simulink model "mrefrobotarm_modified_previous_y_previous_u_previous_ref_cover"  (R2018b)
settings: Solver=FixedStepAuto  StartTime=0.0  StopTime=20  RelTol=1e-3  AbsTol=1e-6
undefined symbols (not defined in the file or in its folder): cc, options
libraries: neural x396, simulink x1
(part 7 of 15)

== system mrefrobotarm_modified_previous_y_previous_u_previous_ref_cover/cov_error/Layer 3/Delays 1 ==
  "p{3}" : Inport  PortDimensions=30
      mask Display: e = 0.06;c1 = [120 230 180]/255;c2 = ([120 230 180]+0)/(256+128);c3 = ([120 230 180]+128)/(256+128);patch([0 1 1 0],[0 0 1 1],c1);patch([0 1 1 1-e 1-e 0+e],[0 0 1 1-e 0+e 0+e],c2);patch([0 0 1 1-e 0+e 0+e],[0 1 1 1-e 1-e 0+e],c3);plot([0 1 1 0 0],[0 0 1 1 0]);
  mux : Mux  Inputs=1
      mask Display: e = 0.06;c1 = [120 150 230]/255;c2 = ([120 150 230]+0)/383;c3 = ([120 150 230]+128)/383;patch([0 1 1 0],[0 0 1 1],c1);patch([0 1 1 1-e 1-e 0+e],[0 0 1 1-e 0+e 0+e],c2);patch([0 0 1 1-e 0+e 0+e],[0 1 1 1-e 1-e 0+e],c3);plot([0 1 1 0 0],[0 0 1 1 0]);disp('Mux')
  "pd{3,2}" : Outport
      mask Display: e = 0.06;c1 = [120 230 180]/255;c2 = ([120 230 180]+0)/(256+128);c3 = ([120 230 180]+128)/(256+128);patch([0 1 1 0],[0 0 1 1],c1);patch([0 1 1 1-e 1-e 0+e],[0 0 1 1-e 0+e 0+e],c2);patch([0 0 1 1-e 0+e 0+e],[0 1 1 1-e 1-e 0+e],c3);plot([0 1 1 0 0],[0 0 1 1 0]);
  wires:
  "p{3}"/1 -> mux/1
  mux/1 -> "pd{3,2}"/1

== system mrefrobotarm_modified_previous_y_previous_u_previous_ref_cover/cov_error/Layer 3/LW{3,2} ==
  "ad{3,2}" : Inport  PortDimensions=30
      mask Display: e = 0.06;c1 = [120 230 180]/255;c2 = ([120 230 180]+0)/(256+128);c3 = ([120 230 180]+128)/(256+128);patch([0 1 1 0],[0 0 1 1],c1);patch([0 1 1 1-e 1-e 0+e],[0 0 1 1-e 0+e 0+e],c2);patch([0 0 1 1-e 0+e 0+e],[0 1 1 1-e 1-e 0+e],c3);plot([0 1 1 0 0],[0 0 1 1 0]);
  "IW{3,2}(1,:)'" : Constant  Value=[-0.36344223341268999671882511393050663173198699951171875;-0.165155178341810537911982237346819601953029632568359375;0.347615078105802999264284380842582322657108306884765625;-0.30164554186513037326022868001018650829792022705078125;0.2759975456345065136787297888076864182949066162109375;0.2465662292665131427593649959817412309348583221435546875;0.1610224607061102319871537247308879159390926361083984375;-0.1798407133675627711522082563533331267535686492919921875;0.401376049002902191009667376420111395418643951416015625;-0.255050273303427832427558996641892008483409881591796875;0.352349460376939038752652777475304901599884033203125;-0.28687203005856043436239133370690979063510894775390625;-0.1992546066370121937705306436328100971877574920654296875;0.233402441264629001427266530299675650894641876220703125;-0.351246745396703807795546481429482810199260711669921875;-0.27181918807968930007490371281164698302745819091796875;0.2299774014947667810648823660812922753393650054931640625;0.283190968807739140711277059381245635449886322021484375;-0.2497764015090132849739035236780182458460330963134765625;-0.27863248514163230229456758024753071367740631103515625;0.37793893813860679475880033351131714880466461181640625;0.3335131904309964756549788944539614021778106689453125;-0.1504481789124049451178422032171511091291904449462890625;0.2409347112974611626601273428605054505169391632080078125;0.1106042034418963371233957104777800850570201873779296875;0.18259052723765833992075613423367030918598175048828125;-0.178194964093014274197912527597509324550628662109375;-0.232453072978504204915140007869922555983066558837890625;0.12259425656011870009454156615902320481836795806884765625;-0.295313678958903758076104395513539202511310577392578125]
      mask Display: e = 0.06;c1 = [120 150 230]/255;c2 = ([120 150 230]+0)/383;c3 = ([120 150 230]+128)/383;patch([0 1 1 0],[0 0 1 1],c1);patch([0 1 1 1-e 1-e 0+e],[0 0 1 1-e 0+e 0+e],c2);patch([0 0 1 1-e 0+e 0+e],[0 1 1 1-e 1-e 0+e],c3);plot([0 1 1 0 0],[0 0 1 1 0]);disp('weights');
  Mux : Mux  Inputs=1
      mask Display: e = 0.06;c1 = [120 150 230]/255;c2 = ([120 150 230]+0)/383;c3 = ([120 150 230]+128)/383;patch([0 1 1 0],[0 0 1 1],c1);patch([0 1 1 1-e 1-e 0+e],[0 0 1 1-e 0+e 0+e],c2);patch([0 0 1 1-e 0+e 0+e],[0 1 1 1-e 1-e 0+e],c3);plot([0 1 1 0 0],[0 0 1 1 0]);disp('Mux');
  dotprod1 : neural/Weight Functions/dotprod
  "lz{3,2}" : Outport
      mask Display: e = 0.06;c1 = [120 230 180]/255;c2 = ([120 230 180]+0)/(256+128);c3 = ([120 230 180]+128)/(256+128);patch([0 1 1 0],[0 0 1 1],c1);patch([0 1 1 1-e 1-e 0+e],[0 0 1 1-e 0+e 0+e],c2);patch([0 0 1 1-e 0+e 0+e],[0 1 1 1-e 1-e 0+e],c3);plot([0 1 1 0 0],[0 0 1 1 0]);
  wires:
  "IW{3,2}(1,:)'"/1 -> dotprod1/1
  "ad{3,2}"/1 -> dotprod1/2
  dotprod1/1 -> Mux/1
  Mux/1 -> "lz{3,2}"/1

== system mrefrobotarm_modified_previous_y_previous_u_previous_ref_cover/cov_no_error/Layer 1/Delays 1 ==
  "p{1}" : Inport  PortDimensions=10
      mask Display: e = 0.06;c1 = [120 230 180]/255;c2 = ([120 230 180]+0)/(256+128);c3 = ([120 230 180]+128)/(256+128);patch([0 1 1 0],[0 0 1 1],c1);patch([0 1 1 1-e 1-e 0+e],[0 0 1 1-e 0+e 0+e],c2);patch([0 0 1 1-e 0+e 0+e],[0 1 1 1-e 1-e 0+e],c3);plot([0 1 1 0 0],[0 0 1 1 0]);
  mux : Mux  Inputs=1
      mask Display: e = 0.06;c1 = [120 150 230]/255;c2 = ([120 150 230]+0)/383;c3 = ([120 150 230]+128)/383;patch([0 1 1 0],[0 0 1 1],c1);patch([0 1 1 1-e 1-e 0+e],[0 0 1 1-e 0+e 0+e],c2);patch([0 0 1 1-e 0+e 0+e],[0 1 1 1-e 1-e 0+e],c3);plot([0 1 1 0 0],[0 0 1 1 0]);disp('Mux')
  "pd{1,1}" : Outport
      mask Display: e = 0.06;c1 = [120 230 180]/255;c2 = ([120 230 180]+0)/(256+128);c3 = ([120 230 180]+128)/(256+128);patch([0 1 1 0],[0 0 1 1],c1);patch([0 1 1 1-e 1-e 0+e],[0 0 1 1-e 0+e 0+e],c2);patch([0 0 1 1-e 0+e 0+e],[0 1 1 1-e 1-e 0+e],c3);plot([0 1 1 0 0],[0 0 1 1 0]);
  wires:
  "p{1}"/1 -> mux/1
  mux/1 -> "pd{1,1}"/1

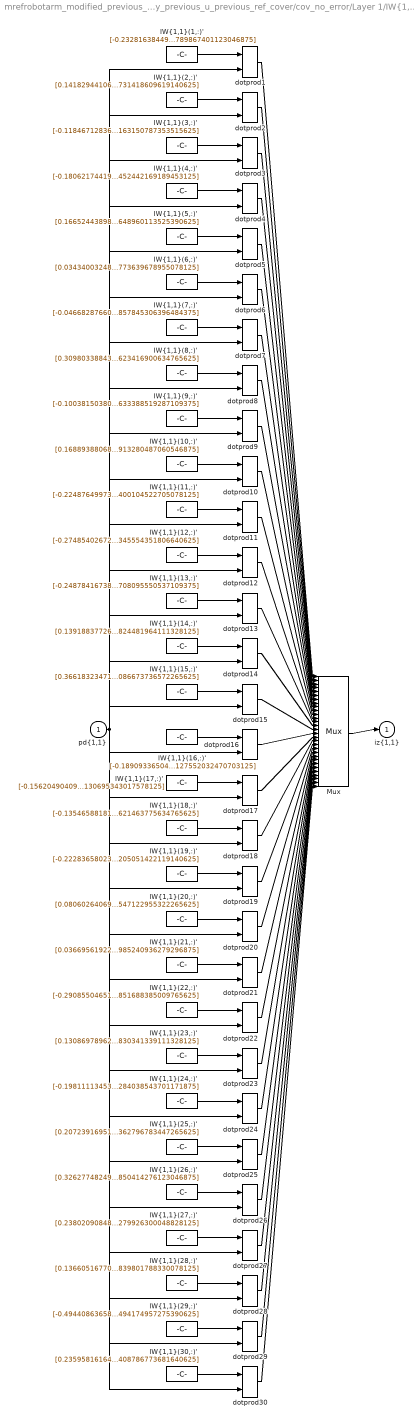
== system mrefrobotarm_modified_previous_y_previous_u_previous_ref_cover/cov_no_error/Layer 1/IW{1,1} ==
  "pd{1,1}" : Inport  PortDimensions=10
      mask Display: e = 0.06;c1 = [120 230 180]/255;c2 = ([120 230 180]+0)/(256+128);c3 = ([120 230 180]+128)/(256+128);patch([0 1 1 0],[0 0 1 1],c1);patch([0 1 1 1-e 1-e 0+e],[0 0 1 1-e 0+e 0+e],c2);patch([0 0 1 1-e 0+e 0+e],[0 1 1 1-e 1-e 0+e],c3);plot([0 1 1 0 0],[0 0 1 1 0]);
  "IW{1,1}(1,:)'" : Constant  Value=[-0.232816384495200312532148245736607350409030914306640625;0.2179398576270096532514486398213193751871585845947265625;0.00979758874001440162315734738740502507425844669342041015625;0.07759532278351477518896217588917352259159088134765625;-0.03578296109490484988580050185191794298589229583740234375;-0.134068358484331573432513096122420392930507659912109375;0.3184571702963874262337640175246633589267730712890625;-0.2184598629676884062877917358491686172783374786376953125;0.11848239573910053501482053661675308831036090850830078125;-0.256553967329338827862983407612773589789867401123046875]
      mask Display: e = 0.06;c1 = [120 150 230]/255;c2 = ([120 150 230]+0)/383;c3 = ([120 150 230]+128)/383;patch([0 1 1 0],[0 0 1 1],c1);patch([0 1 1 1-e 1-e 0+e],[0 0 1 1-e 0+e 0+e],c2);patch([0 0 1 1-e 0+e 0+e],[0 1 1 1-e 1-e 0+e],c3);plot([0 1 1 0 0],[0 0 1 1 0]);disp('Weights');
  "IW{1,1}(10,:)'" : Constant  Value=[0.1688938806870512454594290829845704138278961181640625;0.381459103364416074466447525992407463490962982177734375;0.30186303507656375710865859218756668269634246826171875;0.480258229465630126497899254900403320789337158203125;-0.12049452173532788912257984748066519387066364288330078125;0.14996431208004412649614778274553827941417694091796875;0.08981073971490845242460210329227265901863574981689453125;-0.240164888239770502043057831542682833969593048095703125;0.1714424161086836317924309014415484853088855743408203125;0.00145190267950599870110106603959820859017781913280487060546875]
      mask Display: e = 0.06;c1 = [120 150 230]/255;c2 = ([120 150 230]+0)/383;c3 = ([120 150 230]+128)/383;patch([0 1 1 0],[0 0 1 1],c1);patch([0 1 1 1-e 1-e 0+e],[0 0 1 1-e 0+e 0+e],c2);patch([0 0 1 1-e 0+e 0+e],[0 1 1 1-e 1-e 0+e],c3);plot([0 1 1 0 0],[0 0 1 1 0]);disp('Weights');
  "IW{1,1}(11,:)'" : Constant  Value=[-0.2248764997392367348538755322806537151336669921875;0.41105410405491060732430241841939277946949005126953125;0.1657234394246878406153911100773257203400135040283203125;0.1077899832639681865220637746460852213203907012939453125;-0.1543348784448496935350902958816732279956340789794921875;0.07131387320506217541993265740529750473797321319580078125;0.2162704421912603758304527445943676866590976715087890625;-0.07994022352115277840756135674382676370441913604736328125;0.248269418033737865325605298494338057935237884521484375;0.1716023516014779648486410223995335400104522705078125]
      mask Display: e = 0.06;c1 = [120 150 230]/255;c2 = ([120 150 230]+0)/383;c3 = ([120 150 230]+128)/383;patch([0 1 1 0],[0 0 1 1],c1);patch([0 1 1 1-e 1-e 0+e],[0 0 1 1-e 0+e 0+e],c2);patch([0 0 1 1-e 0+e 0+e],[0 1 1 1-e 1-e 0+e],c3);plot([0 1 1 0 0],[0 0 1 1 0]);disp('Weights');
  "IW{1,1}(12,:)'" : Constant  Value=[-0.274854026724365596567878355926950462162494659423828125;0.2300230565954914097037686815383494831621646881103515625;-0.2464439024372664654993769772772793658077716827392578125;-0.1282591197360603008092994059552438557147979736328125;0.0284855327076480764614263563316853833384811878204345703125;-0.279915672767833967338191314411233179271221160888671875;0.03095000828018605598668244738291832618415355682373046875;0.32448044570328982150186902799759991466999053955078125;-0.0357447986095571490494648969615809619426727294921875;0.086327022995791313775271191843785345554351806640625]
      mask Display: e = 0.06;c1 = [120 150 230]/255;c2 = ([120 150 230]+0)/383;c3 = ([120 150 230]+128)/383;patch([0 1 1 0],[0 0 1 1],c1);patch([0 1 1 1-e 1-e 0+e],[0 0 1 1-e 0+e 0+e],c2);patch([0 0 1 1-e 0+e 0+e],[0 1 1 1-e 1-e 0+e],c3);plot([0 1 1 0 0],[0 0 1 1 0]);disp('Weights');
  "IW{1,1}(13,:)'" : Constant  Value=[-0.2487841673885483328998446950208744965493679046630859375;-0.245428503132846753675977424791199155151844024658203125;-0.309920120905150586754217556517687626183032989501953125;0.10019896818674069172150353779215947724878787994384765625;0.374507443083456015298082775188959203660488128662109375;0.191056862320351406037133301651920191943645477294921875;0.4702083048599126069433395969099365174770355224609375;0.53803390833241138135889514160226099193096160888671875;-0.1869220978197012883459393606244702823460102081298828125;-0.048019763343509901110106596888726926408708095550537109375]
      mask Display: e = 0.06;c1 = [120 150 230]/255;c2 = ([120 150 230]+0)/383;c3 = ([120 150 230]+128)/383;patch([0 1 1 0],[0 0 1 1],c1);patch([0 1 1 1-e 1-e 0+e],[0 0 1 1-e 0+e 0+e],c2);patch([0 0 1 1-e 0+e 0+e],[0 1 1 1-e 1-e 0+e],c3);plot([0 1 1 0 0],[0 0 1 1 0]);disp('Weights');
  "IW{1,1}(14,:)'" : Constant  Value=[0.1391883772688109477400075775221921503543853759765625;0.06629369904048183770317592689025332219898700714111328125;-0.1011387894109859464375489324083901010453701019287109375;-0.11699041710241707414663636654950096271932125091552734375;-0.243529856729322868869047624684753827750682830810546875;0.33130411617758526165999910517712123692035675048828125;0.0137043188173427143983218456924078054726123809814453125;-0.2011655573259559515175709520917735062539577484130859375;0.213554295354308865118042604080983437597751617431640625;0.276335963455466515625857937266118824481964111328125]
      mask Display: e = 0.06;c1 = [120 150 230]/255;c2 = ([120 150 230]+0)/383;c3 = ([120 150 230]+128)/383;patch([0 1 1 0],[0 0 1 1],c1);patch([0 1 1 1-e 1-e 0+e],[0 0 1 1-e 0+e 0+e],c2);patch([0 0 1 1-e 0+e 0+e],[0 1 1 1-e 1-e 0+e],c3);plot([0 1 1 0 0],[0 0 1 1 0]);disp('Weights');
  "IW{1,1}(15,:)'" : Constant  Value=[0.3661832347178719526681334173190407454967498779296875;0.174995375637424455117496790990117006003856658935546875;-0.305173244004664223627543151451391167938709259033203125;0.2241865581074030944197517101201810874044895172119140625;-0.25341912003776989603665015238220803439617156982421875;-0.389938089526184417099585743926581926643848419189453125;-0.10932688953576137624867925524085876531898975372314453125;-0.173230682500792820821544637510669417679309844970703125;-0.09167358048760287925205147985252551734447479248046875;-0.25748585571395443682973791510448791086673736572265625]
      mask Display: e = 0.06;c1 = [120 150 230]/255;c2 = ([120 150 230]+0)/383;c3 = ([120 150 230]+128)/383;patch([0 1 1 0],[0 0 1 1],c1);patch([0 1 1 1-e 1-e 0+e],[0 0 1 1-e 0+e 0+e],c2);patch([0 0 1 1-e 0+e 0+e],[0 1 1 1-e 1-e 0+e],c3);plot([0 1 1 0 0],[0 0 1 1 0]);disp('Weights');
  "IW{1,1}(16,:)'" : Constant  Value=[-0.1890933650459429571366598565873573534190654754638671875;0.390051027170464637006119801299064420163631439208984375;-0.16926823733951312789258736302144825458526611328125;-0.1776784488000019701647858028081827796995639801025390625;0.166930352874170739863046719619887880980968475341796875;-0.049057250337166603826322130998960346914827823638916015625;-0.041501119620162861545420440734233125112950801849365234375;-0.333912429769706642357363080009236000478267669677734375;-0.22428932497446130156504295882768929004669189453125;-0.0218532542813696661898603679219377227127552032470703125]
      mask Display: e = 0.06;c1 = [120 150 230]/255;c2 = ([120 150 230]+0)/383;c3 = ([120 150 230]+128)/383;patch([0 1 1 0],[0 0 1 1],c1);patch([0 1 1 1-e 1-e 0+e],[0 0 1 1-e 0+e 0+e],c2);patch([0 0 1 1-e 0+e 0+e],[0 1 1 1-e 1-e 0+e],c3);plot([0 1 1 0 0],[0 0 1 1 0]);disp('Weights');
  "IW{1,1}(17,:)'" : Constant  Value=[-0.156204904096911290078963929772726260125637054443359375;-0.264618859135635486889981393687776289880275726318359375;-0.446140294613559473813069189418456517159938812255859375;-0.040868645741518626335331276777651510201394557952880859375;-0.06081374496757330216922809995594434440135955810546875;-0.30292739604561347288580464010010473430156707763671875;0.07057474582999682943817987279544468037784099578857421875;-0.16380304878358853404307637902093119919300079345703125;0.28220572883160965904636441337061114609241485595703125;-0.04022463483786938021058432468635146506130695343017578125]
      mask Display: e = 0.06;c1 = [120 150 230]/255;c2 = ([120 150 230]+0)/383;c3 = ([120 150 230]+128)/383;patch([0 1 1 0],[0 0 1 1],c1);patch([0 1 1 1-e 1-e 0+e],[0 0 1 1-e 0+e 0+e],c2);patch([0 0 1 1-e 0+e 0+e],[0 1 1 1-e 1-e 0+e],c3);plot([0 1 1 0 0],[0 0 1 1 0]);disp('Weights');
  "IW{1,1}(18,:)'" : Constant  Value=[-0.13546588181742114098682350231683813035488128662109375;-0.02939553613653468622235465090852812863886356353759765625;-0.336147363930791975850098651790176518261432647705078125;-0.31966394488679394925156884710304439067840576171875;-0.3215969914373226767878577447845600545406341552734375;-0.1902436542887882831021073570809676311910152435302734375;-0.33113436908687143844787215130054391920566558837890625;-0.39157783561824344165103184423060156404972076416015625;0.1413864398116242704350753456310485489666461944580078125;-0.038272862332865677237325741089080111123621463775634765625]
      mask Display: e = 0.06;c1 = [120 150 230]/255;c2 = ([120 150 230]+0)/383;c3 = ([120 150 230]+128)/383;patch([0 1 1 0],[0 0 1 1],c1);patch([0 1 1 1-e 1-e 0+e],[0 0 1 1-e 0+e 0+e],c2);patch([0 0 1 1-e 0+e 0+e],[0 1 1 1-e 1-e 0+e],c3);plot([0 1 1 0 0],[0 0 1 1 0]);disp('Weights');
  "IW{1,1}(19,:)'" : Constant  Value=[-0.2228365802343444113109427462404710240662097930908203125;0.221132410028265169454897431933204643428325653076171875;0.1432822566213183546057763351200264878571033477783203125;-0.154286973287174056235215857668663375079631805419921875;-0.2389845744478707179059284726463374681770801544189453125;0.07427667026116148429881747006220393814146518707275390625;0.152309043555764411781439093829249031841754913330078125;-0.158159403129818632027792091321316547691822052001953125;-0.321803318052325926235113229267881251871585845947265625;0.331994217610607267321398694548406638205051422119140625]
      mask Display: e = 0.06;c1 = [120 150 230]/255;c2 = ([120 150 230]+0)/383;c3 = ([120 150 230]+128)/383;patch([0 1 1 0],[0 0 1 1],c1);patch([0 1 1 1-e 1-e 0+e],[0 0 1 1-e 0+e 0+e],c2);patch([0 0 1 1-e 0+e 0+e],[0 1 1 1-e 1-e 0+e],c3);plot([0 1 1 0 0],[0 0 1 1 0]);disp('Weights');
  "IW{1,1}(2,:)'" : Constant  Value=[0.1418294410694424800833957078793901018798351287841796875;0.2163596747671927833511773542340961284935474395751953125;0.006673786734878991121211466719387317425571382045745849609375;0.125332803321089703008084370594588108360767364501953125;0.2236668593030913532171410906812525354325771331787109375;0.06416405555974562247012471516427467577159404754638671875;0.30314211911453525782889073525439016520977020263671875;0.3763140102963100641630944664939306676387786865234375;0.281611720838433055025262774506700225174427032470703125;0.006654770573335945516024736434701480902731418609619140625]
      mask Display: e = 0.06;c1 = [120 150 230]/255;c2 = ([120 150 230]+0)/383;c3 = ([120 150 230]+128)/383;patch([0 1 1 0],[0 0 1 1],c1);patch([0 1 1 1-e 1-e 0+e],[0 0 1 1-e 0+e 0+e],c2);patch([0 0 1 1-e 0+e 0+e],[0 1 1 1-e 1-e 0+e],c3);plot([0 1 1 0 0],[0 0 1 1 0]);disp('Weights');
  "IW{1,1}(20,:)'" : Constant  Value=[0.0806026406933142147703819091475452296435832977294921875;-0.306285227886031241606445973957306705415248870849609375;-0.18366994302208217160199410500354133546352386474609375;-0.2198604928822714132952143017973867245018482208251953125;-0.2231519653798757774065819603492855094373226165771484375;0.09645373460015672917311491119107813574373722076416015625;0.164281010938679028487996447438490577042102813720703125;-0.3200685795055464577529846792458556592464447021484375;0.1621835307111210988662008958272053860127925872802734375;-0.1713450738891130475938240351752028800547122955322265625]
      mask Display: e = 0.06;c1 = [120 150 230]/255;c2 = ([120 150 230]+0)/383;c3 = ([120 150 230]+128)/383;patch([0 1 1 0],[0 0 1 1],c1);patch([0 1 1 1-e 1-e 0+e],[0 0 1 1-e 0+e 0+e],c2);patch([0 0 1 1-e 0+e 0+e],[0 1 1 1-e 1-e 0+e],c3);plot([0 1 1 0 0],[0 0 1 1 0]);disp('Weights');
  "IW{1,1}(21,:)'" : Constant  Value=[0.03669561922376436691184409255583886988461017608642578125;-0.413492761556377264042794195120222866535186767578125;0.1937476095665302266990437374261091463267803192138671875;-0.2953156414632742698955780724645592272281646728515625;-0.1703157205887977365676988483755849301815032958984375;0.302215909969603735429899415976251475512981414794921875;0.1621722263023846200002964224040624685585498809814453125;-0.018732372452806435314531796620940440334379673004150390625;0.216300659030234265767234091981663368642330169677734375;-0.0289332479865664626839105721956002525985240936279296875]
      mask Display: e = 0.06;c1 = [120 150 230]/255;c2 = ([120 150 230]+0)/383;c3 = ([120 150 230]+128)/383;patch([0 1 1 0],[0 0 1 1],c1);patch([0 1 1 1-e 1-e 0+e],[0 0 1 1-e 0+e 0+e],c2);patch([0 0 1 1-e 0+e 0+e],[0 1 1 1-e 1-e 0+e],c3);plot([0 1 1 0 0],[0 0 1 1 0]);disp('Weights');
  "IW{1,1}(22,:)'" : Constant  Value=[-0.290855046516667214984153133627842180430889129638671875;-0.169708808503639285714115203518304042518138885498046875;-0.05561531108973073733725556166973547078669071197509765625;-0.01051333740893246708469899175497630494646728038787841796875;-0.15836707382769821261803144807345233857631683349609375;0.2791739322138226953029516153037548065185546875;0.287158434133134965460243392953998409211635589599609375;0.0277604612424260759062644154937515850178897380828857421875;0.17361153790517847017582653279532678425312042236328125;-0.110783296897912553191645201877690851688385009765625]
      mask Display: e = 0.06;c1 = [120 150 230]/255;c2 = ([120 150 230]+0)/383;c3 = ([120 150 230]+128)/383;patch([0 1 1 0],[0 0 1 1],c1);patch([0 1 1 1-e 1-e 0+e],[0 0 1 1-e 0+e 0+e],c2);patch([0 0 1 1-e 0+e 0+e],[0 1 1 1-e 1-e 0+e],c3);plot([0 1 1 0 0],[0 0 1 1 0]);disp('Weights');
  "IW{1,1}(23,:)'" : Constant  Value=[0.1308697896224377543727968031816999427974224090576171875;-0.356061926493931035775375448793056420981884002685546875;0.1017050860801818890077896639922983013093471527099609375;0.119719011302845845801101631877827458083629608154296875;-0.291455520695850622825417985950480215251445770263671875;0.492623523089699089094750661388388834893703460693359375;-0.1517316310937479040266140373205416835844516754150390625;-0.1794544948922624783005375093125621788203716278076171875;-0.0258670493679656297858482361107235192321240901947021484375;0.350943705502367919724093781042029149830341339111328125]
      mask Display: e = 0.06;c1 = [120 150 230]/255;c2 = ([120 150 230]+0)/383;c3 = ([120 150 230]+128)/383;patch([0 1 1 0],[0 0 1 1],c1);patch([0 1 1 1-e 1-e 0+e],[0 0 1 1-e 0+e 0+e],c2);patch([0 0 1 1-e 0+e 0+e],[0 1 1 1-e 1-e 0+e],c3);plot([0 1 1 0 0],[0 0 1 1 0]);disp('Weights');
  "IW{1,1}(24,:)'" : Constant  Value=[-0.19811113453014350671566035089199431240558624267578125;0.3222581152191830167197394985123537480831146240234375;-0.2248971416038330062292516231536865234375;-0.21881212676011918549789925236837007105350494384765625;0.08568240252901389297779388698472757823765277862548828125;-0.052799644239780167687126066766722942702472209930419921875;0.30688129749510506538712206747732125222682952880859375;-0.0802967837620946756072015659810858778655529022216796875;0.08592332417998048421647894201669259928166866302490234375;-0.1673975850986572921907935551644186489284038543701171875]
      mask Display: e = 0.06;c1 = [120 150 230]/255;c2 = ([120 150 230]+0)/383;c3 = ([120 150 230]+128)/383;patch([0 1 1 0],[0 0 1 1],c1);patch([0 1 1 1-e 1-e 0+e],[0 0 1 1-e 0+e 0+e],c2);patch([0 0 1 1-e 0+e 0+e],[0 1 1 1-e 1-e 0+e],c3);plot([0 1 1 0 0],[0 0 1 1 0]);disp('Weights');
  "IW{1,1}(25,:)'" : Constant  Value=[0.2072391695154046364901745391762233339250087738037109375;0.454825828462298187293555429278057999908924102783203125;0.1553650820099924667605506556355976499617099761962890625;0.0729869830792790608153808307179133407771587371826171875;0.264205376797746305239655839613988064229488372802734375;0.31155092672919260099462235302780754864215850830078125;0.142573824703868201613232713498291559517383575439453125;0.0020602921316580473376500748372563975863158702850341796875;0.366396840530492706733411978348158299922943115234375;-0.048368934269253295588075758359991596080362796783447265625]
      mask Display: e = 0.06;c1 = [120 150 230]/255;c2 = ([120 150 230]+0)/383;c3 = ([120 150 230]+128)/383;patch([0 1 1 0],[0 0 1 1],c1);patch([0 1 1 1-e 1-e 0+e],[0 0 1 1-e 0+e 0+e],c2);patch([0 0 1 1-e 0+e 0+e],[0 1 1 1-e 1-e 0+e],c3);plot([0 1 1 0 0],[0 0 1 1 0]);disp('Weights');
  "IW{1,1}(26,:)'" : Constant  Value=[0.326277482499976068108793469946249388158321380615234375;0.08202126981506120684262128861519158817827701568603515625;0.40914149931839871587868628921569325029850006103515625;0.1235879391668728566333612661765073426067829132080078125;0.0307358575801956017403693266487607615999877452850341796875;-0.12672241717916710168623239951557479798793792724609375;-0.1957018649578968483293550661983317695558071136474609375;0.042429450574601408618935494132529129274189472198486328125;-0.191397940511998487789213641008245758712291717529296875;0.112936610515262880749531859692069701850414276123046875]
      mask Display: e = 0.06;c1 = [120 150 230]/255;c2 = ([120 150 230]+0)/383;c3 = ([120 150 230]+128)/383;patch([0 1 1 0],[0 0 1 1],c1);patch([0 1 1 1-e 1-e 0+e],[0 0 1 1-e 0+e 0+e],c2);patch([0 0 1 1-e 0+e 0+e],[0 1 1 1-e 1-e 0+e],c3);plot([0 1 1 0 0],[0 0 1 1 0]);disp('Weights');
  "IW{1,1}(27,:)'" : Constant  Value=[0.2380209084838374178350051124652964062988758087158203125;-0.25234459075706894282120629213750362396240234375;0.04029507721190740687777775974609539844095706939697265625;-0.1849313431100750582114500275565660558640956878662109375;-0.02542071997715251996385887878204812295734882354736328125;0.2487714630258091863534986032391316257417201995849609375;0.1319644188429672515550095113212591968476772308349609375;-0.0785779966407837704434058423430542461574077606201171875;0.047603046342789841205433987170181353576481342315673828125;-0.30315767282660843751074253304977901279926300048828125]
      mask Display: e = 0.06;c1 = [120 150 230]/255;c2 = ([120 150 230]+0)/383;c3 = ([120 150 230]+128)/383;patch([0 1 1 0],[0 0 1 1],c1);patch([0 1 1 1-e 1-e 0+e],[0 0 1 1-e 0+e 0+e],c2);patch([0 0 1 1-e 0+e 0+e],[0 1 1 1-e 1-e 0+e],c3);plot([0 1 1 0 0],[0 0 1 1 0]);disp('Weights');
  "IW{1,1}(28,:)'" : Constant  Value=[0.136605167705069308059506738572963513433933258056640625;-0.10123138913781259962121339412988163530826568603515625;-0.0172616637220188266776954577608194085769355297088623046875;-0.1003700761539133290423109201583429239690303802490234375;-0.0678402671941051582660264784863102249801158905029296875;0.11916269568666328082517935627038241364061832427978515625;-0.346494939272794066909000321174971759319305419921875;0.275695945511745865719177572827902622520923614501953125;-0.332567429851041762578489624502253718674182891845703125;0.2245339650803064579509538134516333229839801788330078125]
      mask Display: e = 0.06;c1 = [120 150 230]/255;c2 = ([120 150 230]+0)/383;c3 = ([120 150 230]+128)/383;patch([0 1 1 0],[0 0 1 1],c1);patch([0 1 1 1-e 1-e 0+e],[0 0 1 1-e 0+e 0+e],c2);patch([0 0 1 1-e 0+e 0+e],[0 1 1 1-e 1-e 0+e],c3);plot([0 1 1 0 0],[0 0 1 1 0]);disp('Weights');
  "IW{1,1}(29,:)'" : Constant  Value=[-0.4944086365862669918413985215011052787303924560546875;-0.55424579803283080536857596598565578460693359375;-0.342223614581396218259357056012959219515323638916015625;-0.0351502192926707868192437445031828247010707855224609375;-0.0973742607049431774246528448202298022806644439697265625;-0.0209730185931580569158594329337574890814721584320068359375;-0.34378718573028288485460279844119213521480560302734375;-0.263185956779630692015103932135389186441898345947265625;-0.13753087290669097075834770294022746384143829345703125;-0.0361110684343338983470772518558078445494174957275390625]
      mask Display: e = 0.06;c1 = [120 150 230]/255;c2 = ([120 150 230]+0)/383;c3 = ([120 150 230]+128)/383;patch([0 1 1 0],[0 0 1 1],c1);patch([0 1 1 1-e 1-e 0+e],[0 0 1 1-e 0+e 0+e],c2);patch([0 0 1 1-e 0+e 0+e],[0 1 1 1-e 1-e 0+e],c3);plot([0 1 1 0 0],[0 0 1 1 0]);disp('Weights');
  "IW{1,1}(3,:)'" : Constant  Value=[-0.118467128369881880001202034691232256591320037841796875;0.14509175670659424373099000149522908031940460205078125;-0.2364524329857893569784010878720437176525592803955078125;-0.04745728828579258429254394968666019849479198455810546875;0.06976195967193542235573744392240769229829311370849609375;0.1899442015700345820494732151928474195301532745361328125;-0.1360815627507493130732285635531297884881496429443359375;-0.198365622741620450941724129734211601316928863525390625;-0.23332389544343146159377511139609850943088531494140625;-0.04085166162289612101776725694435299374163150787353515625]
      mask Display: e = 0.06;c1 = [120 150 230]/255;c2 = ([120 150 230]+0)/383;c3 = ([120 150 230]+128)/383;patch([0 1 1 0],[0 0 1 1],c1);patch([0 1 1 1-e 1-e 0+e],[0 0 1 1-e 0+e 0+e],c2);patch([0 0 1 1-e 0+e 0+e],[0 1 1 1-e 1-e 0+e],c3);plot([0 1 1 0 0],[0 0 1 1 0]);disp('Weights');
  "IW{1,1}(30,:)'" : Constant  Value=[0.23595816164212013443801652101683430373668670654296875;-0.0971950739796785534441170284480904228985309600830078125;0.13562425954600432209673499528435058891773223876953125;-0.25851468762828933023456556838937103748321533203125;-0.178064718336138627652331933859386481344699859619140625;-0.1322485165484958147263938599280663765966892242431640625;-0.308813374631858372776349597188527695834636688232421875;-0.357359439300734715860841106405132450163364410400390625;-0.03494929717273616287531723401116323657333850860595703125;0.023790716863915963019682209278471418656408786773681640625]
      mask Display: e = 0.06;c1 = [120 150 230]/255;c2 = ([120 150 230]+0)/383;c3 = ([120 150 230]+128)/383;patch([0 1 1 0],[0 0 1 1],c1);patch([0 1 1 1-e 1-e 0+e],[0 0 1 1-e 0+e 0+e],c2);patch([0 0 1 1-e 0+e 0+e],[0 1 1 1-e 1-e 0+e],c3);plot([0 1 1 0 0],[0 0 1 1 0]);disp('Weights');
  "IW{1,1}(4,:)'" : Constant  Value=[-0.18062174419628707067175810152548365294933319091796875;-0.115172514893159994020521708080195821821689605712890625;0.192600373914811939801694506968487985432147979736328125;-0.16136071333539570016313291489495895802974700927734375;-0.01506989005102719707263059234492175164632499217987060546875;-0.261061656989213408674999072900391183793544769287109375;-0.21756725260179032854779279659851454198360443115234375;-0.058048608226782004437804829422020702622830867767333984375;0.003578499493176907041147583043994018225930631160736083984375;0.285928214507425781931715391692705452442169189453125]
      mask Display: e = 0.06;c1 = [120 150 230]/255;c2 = ([120 150 230]+0)/383;c3 = ([120 150 230]+128)/383;patch([0 1 1 0],[0 0 1 1],c1);patch([0 1 1 1-e 1-e 0+e],[0 0 1 1-e 0+e 0+e],c2);patch([0 0 1 1-e 0+e 0+e],[0 1 1 1-e 1-e 0+e],c3);plot([0 1 1 0 0],[0 0 1 1 0]);disp('Weights');
  "IW{1,1}(5,:)'" : Constant  Value=[0.16652443898008917333442013841704465448856353759765625;-0.186300343694521808313169231041683815419673919677734375;0.32265665592481551637860093251219950616359710693359375;-0.035761178123781094118083245803063618950545787811279296875;-0.1570134332029285706422427892903215251863002777099609375;-0.043408754489405405874169474600421381182968616485595703125;0.050528833807064237049200272622329066507518291473388671875;-0.08992444083225627216027220356409088708460330963134765625;0.282324868374548787475220024134614504873752593994140625;0.2365809680935627989928349279580288566648960113525390625]
      mask Display: e = 0.06;c1 = [120 150 230]/255;c2 = ([120 150 230]+0)/383;c3 = ([120 150 230]+128)/383;patch([0 1 1 0],[0 0 1 1],c1);patch([0 1 1 1-e 1-e 0+e],[0 0 1 1-e 0+e 0+e],c2);patch([0 0 1 1-e 0+e 0+e],[0 1 1 1-e 1-e 0+e],c3);plot([0 1 1 0 0],[0 0 1 1 0]);disp('Weights');
  "IW{1,1}(6,:)'" : Constant  Value=[0.034340032480570277517717414639264461584389209747314453125;-0.258418189516405771843921002073329873383045196533203125;-0.34267281701603591326232844949117861688137054443359375;0.1443087558341543952256103011677623726427555084228515625;0.191619695311630200418306912979460321366786956787109375;0.2041806719881093801216564997957902960479259490966796875;-0.0306477286103419670204583979966628248803317546844482421875;0.292317393636743805274136320804245769977569580078125;0.0659958420873447415555546058385516516864299774169921875;-0.221349042492399228354571505406056530773639678955078125]
      mask Display: e = 0.06;c1 = [120 150 230]/255;c2 = ([120 150 230]+0)/383;c3 = ([120 150 230]+128)/383;patch([0 1 1 0],[0 0 1 1],c1);patch([0 1 1 1-e 1-e 0+e],[0 0 1 1-e 0+e 0+e],c2);patch([0 0 1 1-e 0+e 0+e],[0 1 1 1-e 1-e 0+e],c3);plot([0 1 1 0 0],[0 0 1 1 0]);disp('Weights');
  "IW{1,1}(7,:)'" : Constant  Value=[-0.046682876607548169645145463846347411163151264190673828125;0.11309677820304787909666544010178768076002597808837890625;0.137312000674695955382276224554516375064849853515625;-0.1039939044379677712814924461781629361212253570556640625;-0.2799768091829812899362650568946264684200286865234375;0.182364446259938695060753843790735118091106414794921875;0.2499384891907307781888647468804265372455120086669921875;-0.136441052789205874429256937219179235398769378662109375;-0.169732922802202923495684672161587513983249664306640625;-0.054557323715807092001650602242079912684857845306396484375]
      mask Display: e = 0.06;c1 = [120 150 230]/255;c2 = ([120 150 230]+0)/383;c3 = ([120 150 230]+128)/383;patch([0 1 1 0],[0 0 1 1],c1);patch([0 1 1 1-e 1-e 0+e],[0 0 1 1-e 0+e 0+e],c2);patch([0 0 1 1-e 0+e 0+e],[0 1 1 1-e 1-e 0+e],c3);plot([0 1 1 0 0],[0 0 1 1 0]);disp('Weights');
  "IW{1,1}(8,:)'" : Constant  Value=[0.30980338843371379997648773496621288359165191650390625;-0.053564283320576812352786788551384233869612216949462890625;0.1747634380908723306102814376572496257722377777099609375;0.3515608122318465422750932702911086380481719970703125;-0.014224394472559305502290527556397137232124805450439453125;-0.1207513111979061637413224161718972027301788330078125;-0.244733028704410049414263994549401104450225830078125;0.2254633955359826302800030362050165422260761260986328125;0.1835163994520099539631274865314480848610401153564453125;-0.01695995874979806805615822895560995675623416900634765625]
      mask Display: e = 0.06;c1 = [120 150 230]/255;c2 = ([120 150 230]+0)/383;c3 = ([120 150 230]+128)/383;patch([0 1 1 0],[0 0 1 1],c1);patch([0 1 1 1-e 1-e 0+e],[0 0 1 1-e 0+e 0+e],c2);patch([0 0 1 1-e 0+e 0+e],[0 1 1 1-e 1-e 0+e],c3);plot([0 1 1 0 0],[0 0 1 1 0]);disp('Weights');
  "IW{1,1}(9,:)'" : Constant  Value=[-0.100381503809379657443656697068945504724979400634765625;-0.0669162080276439752424266771413385868072509765625;0.264898755967136689815077943421783857047557830810546875;0.1055622065280745480730928420598502270877361297607421875;0.211003741368687602886211607255972921848297119140625;-0.11260445611176074509618416641387739218771457672119140625;-0.27850079376451863932828700853860937058925628662109375;0.04331611820108628718717369565638364292681217193603515625;-0.408010237993691016189501397093408741056919097900390625;0.021796270875222532870107983171692467294633388519287109375]
      mask Display: e = 0.06;c1 = [120 150 230]/255;c2 = ([120 150 230]+0)/383;c3 = ([120 150 230]+128)/383;patch([0 1 1 0],[0 0 1 1],c1);patch([0 1 1 1-e 1-e 0+e],[0 0 1 1-e 0+e 0+e],c2);patch([0 0 1 1-e 0+e 0+e],[0 1 1 1-e 1-e 0+e],c3);plot([0 1 1 0 0],[0 0 1 1 0]);disp('Weights');
  Mux : Mux  Inputs=30
      mask Display: e = 0.06;c1 = [120 150 230]/255;c2 = ([120 150 230]+0)/383;c3 = ([120 150 230]+128)/383;patch([0 1 1 0],[0 0 1 1],c1);patch([0 1 1 1-e 1-e 0+e],[0 0 1 1-e 0+e 0+e],c2);patch([0 0 1 1-e 0+e 0+e],[0 1 1 1-e 1-e 0+e],c3);plot([0 1 1 0 0],[0 0 1 1 0]);disp('Mux');
  dotprod{1..30} (30 alike) : neural/Weight Functions/dotprod
  "iz{1,1}" : Outport
      mask Display: e = 0.06;c1 = [120 230 180]/255;c2 = ([120 230 180]+0)/(256+128);c3 = ([120 230 180]+128)/(256+128);patch([0 1 1 0],[0 0 1 1],c1);patch([0 1 1 1-e 1-e 0+e],[0 0 1 1-e 0+e 0+e],c2);patch([0 0 1 1-e 0+e 0+e],[0 1 1 1-e 1-e 0+e],c3);plot([0 1 1 0 0],[0 0 1 1 0]);
  wires:
  "IW{1,1}(1,:)'"/1 -> dotprod1/1
  "pd{1,1}"/1 -> dotprod1/2, dotprod2/2, dotprod3/2, dotprod4/2, dotprod5/2, dotprod6/2, dotprod7/2, dotprod8/2, dotprod9/2, dotprod10/2, dotprod11/2, dotprod12/2, dotprod13/2, dotprod14/2, dotprod15/2, dotprod16/2, dotprod17/2, dotprod18/2, dotprod19/2, dotprod20/2, dotprod21/2, dotprod22/2, dotprod23/2, dotprod24/2, dotprod25/2, dotprod26/2, dotprod27/2, dotprod28/2, dotprod29/2, dotprod30/2
  dotprod1/1 -> Mux/1
  "IW{1,1}(2,:)'"/1 -> dotprod2/1
  dotprod2/1 -> Mux/2
  "IW{1,1}(3,:)'"/1 -> dotprod3/1
  dotprod3/1 -> Mux/3
  "IW{1,1}(4,:)'"/1 -> dotprod4/1
  dotprod4/1 -> Mux/4
  "IW{1,1}(5,:)'"/1 -> dotprod5/1
  dotprod5/1 -> Mux/5
  "IW{1,1}(6,:)'"/1 -> dotprod6/1
  dotprod6/1 -> Mux/6
  "IW{1,1}(7,:)'"/1 -> dotprod7/1
  dotprod7/1 -> Mux/7
  "IW{1,1}(8,:)'"/1 -> dotprod8/1
  dotprod8/1 -> Mux/8
  "IW{1,1}(9,:)'"/1 -> dotprod9/1
  dotprod9/1 -> Mux/9
  "IW{1,1}(10,:)'"/1 -> dotprod10/1
  dotprod10/1 -> Mux/10
  "IW{1,1}(11,:)'"/1 -> dotprod11/1
  dotprod11/1 -> Mux/11
  "IW{1,1}(12,:)'"/1 -> dotprod12/1
  dotprod12/1 -> Mux/12
  "IW{1,1}(13,:)'"/1 -> dotprod13/1
  dotprod13/1 -> Mux/13
  "IW{1,1}(14,:)'"/1 -> dotprod14/1
  dotprod14/1 -> Mux/14
  "IW{1,1}(15,:)'"/1 -> dotprod15/1
  dotprod15/1 -> Mux/15
  "IW{1,1}(16,:)'"/1 -> dotprod16/1
  dotprod16/1 -> Mux/16
  "IW{1,1}(17,:)'"/1 -> dotprod17/1
  dotprod17/1 -> Mux/17
  "IW{1,1}(18,:)'"/1 -> dotprod18/1
  dotprod18/1 -> Mux/18
  "IW{1,1}(19,:)'"/1 -> dotprod19/1
  dotprod19/1 -> Mux/19
  "IW{1,1}(20,:)'"/1 -> dotprod20/1
  dotprod20/1 -> Mux/20
  "IW{1,1}(21,:)'"/1 -> dotprod21/1
  dotprod21/1 -> Mux/21
  "IW{1,1}(22,:)'"/1 -> dotprod22/1
  dotprod22/1 -> Mux/22
  "IW{1,1}(23,:)'"/1 -> dotprod23/1
  dotprod23/1 -> Mux/23
  "IW{1,1}(24,:)'"/1 -> dotprod24/1
  dotprod24/1 -> Mux/24
  "IW{1,1}(25,:)'"/1 -> dotprod25/1
  dotprod25/1 -> Mux/25
  "IW{1,1}(26,:)'"/1 -> dotprod26/1
  dotprod26/1 -> Mux/26
  "IW{1,1}(27,:)'"/1 -> dotprod27/1
  dotprod27/1 -> Mux/27
  "IW{1,1}(28,:)'"/1 -> dotprod28/1
  dotprod28/1 -> Mux/28
  "IW{1,1}(29,:)'"/1 -> dotprod29/1
  dotprod29/1 -> Mux/29
  "IW{1,1}(30,:)'"/1 -> dotprod30/1
  dotprod30/1 -> Mux/30
  Mux/1 -> "iz{1,1}"/1

== system mrefrobotarm_modified_previous_y_previous_u_previous_ref_cover/cov_no_error/Layer 2/Delays 1 ==
  "p{2}" : Inport  PortDimensions=30
      mask Display: e = 0.06;c1 = [120 230 180]/255;c2 = ([120 230 180]+0)/(256+128);c3 = ([120 230 180]+128)/(256+128);patch([0 1 1 0],[0 0 1 1],c1);patch([0 1 1 1-e 1-e 0+e],[0 0 1 1-e 0+e 0+e],c2);patch([0 0 1 1-e 0+e 0+e],[0 1 1 1-e 1-e 0+e],c3);plot([0 1 1 0 0],[0 0 1 1 0]);
  mux : Mux  Inputs=1
      mask Display: e = 0.06;c1 = [120 150 230]/255;c2 = ([120 150 230]+0)/383;c3 = ([120 150 230]+128)/383;patch([0 1 1 0],[0 0 1 1],c1);patch([0 1 1 1-e 1-e 0+e],[0 0 1 1-e 0+e 0+e],c2);patch([0 0 1 1-e 0+e 0+e],[0 1 1 1-e 1-e 0+e],c3);plot([0 1 1 0 0],[0 0 1 1 0]);disp('Mux')
  "pd{2,1}" : Outport
      mask Display: e = 0.06;c1 = [120 230 180]/255;c2 = ([120 230 180]+0)/(256+128);c3 = ([120 230 180]+128)/(256+128);patch([0 1 1 0],[0 0 1 1],c1);patch([0 1 1 1-e 1-e 0+e],[0 0 1 1-e 0+e 0+e],c2);patch([0 0 1 1-e 0+e 0+e],[0 1 1 1-e 1-e 0+e],c3);plot([0 1 1 0 0],[0 0 1 1 0]);
  wires:
  "p{2}"/1 -> mux/1
  mux/1 -> "pd{2,1}"/1
